simulink model "Passive_Suspension_System_2018"  (R2018a)
settings: Solver=VariableStepAuto  StartTime=0.0  StopTime=10.0  RelTol=1e-3
settings Model: Creator=99003188  LastModifiedBy=99003188
settings DataIOCC: ReturnWorkspaceOutputs=on
settings SFSimCC: SimUseLocalCustomCode=on
settings RTWCC: RTWUseLocalCustomCode=on

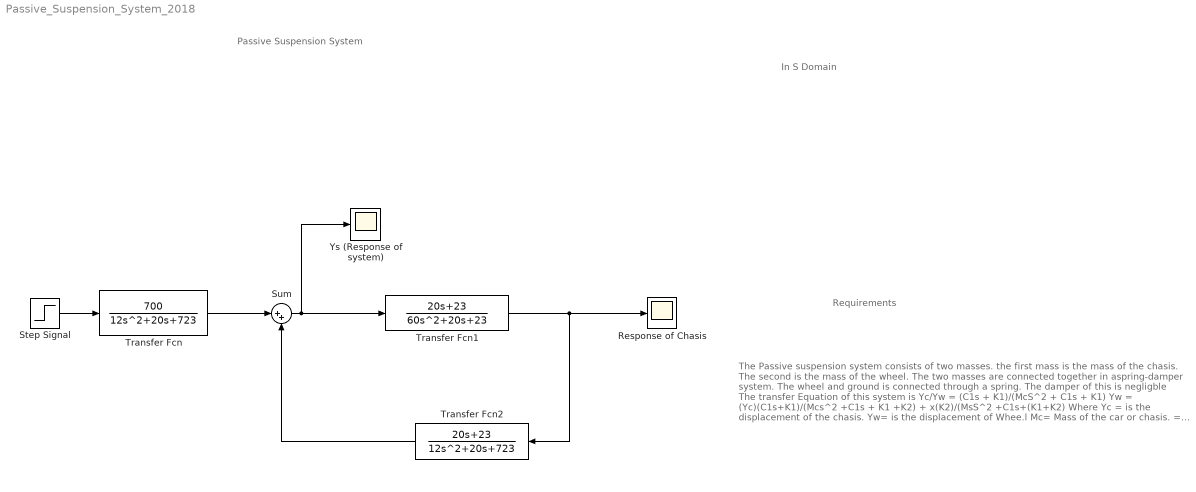
== system Passive_Suspension_System_2018 ==
  note: The Passive suspension system consists of two masses. the first mass is the mass of the chasis. The second is the mass of the wheel. The two masses are connected together in aspring-damper system. The wheel and ground is connected through a spring. The damper of this is negligble
      | The transfer Equation of this system is
      | Yc/Yw = (C1s + K1)/(McS^2 + C1s + K1)
      | Yw = (Yc)(C1s+K1)/(Mcs^2 +C1s + K1 +K2) + x(K2)/(MsS^2 +C1s+(K1+K2)
      | Where
      | Yc = is the displacement of the chasis.
      | Yw= is the displacement of Whee.l
      | Mc= Mass of the car or chasis. = 60 Kg.
      | Mw = Mass of the wheel. = 12 Kg.
      | K1 = Spring coefficent between chasis and wheel = 23 N/mm
      | C1 = damper Coefficent betweem chasis and wheel = 20 Ns/mm.
      | K2 = spring between wheel and ground = 700 N/mm.
  note: In S Domain
  note: Requirements
  note: Passive Suspension System
  Response of Chasis : Scope
  Step Signal : Step  After=30  SampleTime=0
  Sum : Sum  Inputs=|++
  Transfer Fcn : TransferFcn  Numerator=[700]  Denominator=[12 20 723]
  Transfer Fcn1 : TransferFcn  Numerator=[20 23]  Denominator=[60 20 23]
  Transfer Fcn2 : TransferFcn  Numerator=[20 23]  Denominator=[12 20 723]
  Ys (Response of system) : Scope
  wires:
  Transfer Fcn1/1 -> Response of Chasis/1, Transfer Fcn2/1
  Step Signal/1 -> Transfer Fcn/1
  Transfer Fcn/1 -> Sum/1
  Sum/1 -> Transfer Fcn1/1, Ys (Response of system)/1
  Transfer Fcn2/1 -> Sum/2
